simulink subsystem "VehicleElectric"  (R2024b)
settings: Solver=VariableStepAuto  StartTime=0.0  StopTime=10.0  RelTol=1e-3
libraries: nesl_utility x1
Description:
  | Vehicle Electric Architecture
  | 
  | ⚡ Main Features:
  | - Dual motor layout: front motor (EM1) and rear motor (EM2)
  | - Central battery pack supplying HV power to motors and charger
  | - Charger block for external charging interface
  | - Driveline subsystem connects motor torque to wheels
  | - Vehicle-level representation with visual layout
  | 
  | 📤 Outputs: Front/Rear Motor Torque, Battery Power, Driveline Response
  | 
  | 📌 Use Case: Vehicle-level studies of AWD/FWD/RWD configurations, energy flow, and efficiency
settings Model: Creator=jjha  LastModifiedBy=jjha
settings OptimizationCC: ReuseModelBlockBuffer=off
settings RTWCC: GPUComputeCapability=3.5

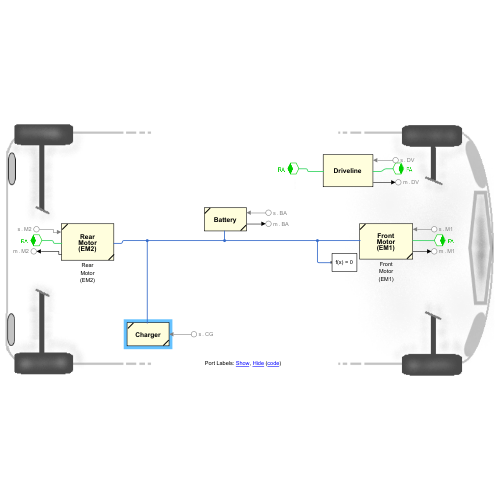
[thumbnail: Simulink's stored preview of the top-level diagram]
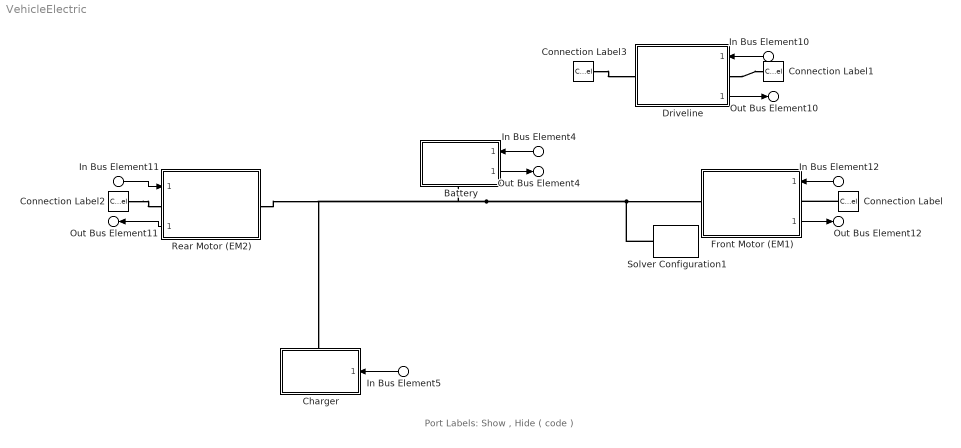
== system VehicleElectric ==
  note: Port Labels: Show , Hide ( code )
  In Bus Element4 : Inport  PortName=s  Element=BA
  In Bus Element10 : Inport  PortName=s  Element=DV
  In Bus Element11 : Inport  PortName=s  Element=M2
  In Bus Element12 : Inport  PortName=s  Element=M1
  In Bus Element5 : Inport  PortName=s  Element=CG
  Battery : Subsystem  ReferencedSubsystem=BatteryLumped
      settings: PortSchema="{\"entries\":[{\"content\":{\"sides\":[{\"content\":{\"connectorIds\":[\"In1\",\"Out1\"]},\"type\":\"ConnectorPlacement.EquallySpacedRectSide\",\"uuid\":\"8937d0fc-2bf4-4b6f-a857-82b384a76c94\"},{\"content\":{\"side\":\"RIGHT\"},\"type\":\"ConnectorPlacement.EquallySpacedRectSide\",\"uuid\":\"1ccbeec6-a013-4076-9f98-cb308866a19c\"},{\"content\":{\"side\":\"TOP\"},\"type\":\"ConnectorPlacement.EquallySpacedRectSide\",\"uuid\":\"77a454e3-c37c-480e-9dd0-9550186f5eb3\"},{\"content\":{\"connectorIds\":[\"RConn1\"],\"side\":\"BOTTOM\"},\"type\":\"ConnectorPlacement.EquallySpacedRectSide\",\"uuid\":\"f9a87c6a-7374-41c2-a5df-89d60c915a70\"}]},\"type\":\"ConnectorPlacement.EquallySpacedConnector\",\"uuid\":\"fe008494-fd6d-45a8-bf6b-36872afbad95\"}],\"packageUris\":[\"http://schema.mathworks.com/mf0/Connector/R2020b\"],\"version\":\"1.0\"}"
  Charger : Subsystem  ReferencedSubsystem=Charger
      settings: PortSchema="{\"entries\":[{\"content\":{\"sides\":[{\"content\":{\"connectorIds\":[\"In1\"]},\"type\":\"ConnectorPlacement.EquallySpacedRectSide\",\"uuid\":\"cb45011f-5d5d-4b7e-92e7-7d115d1e4fd6\"},{\"content\":{\"side\":\"RIGHT\"},\"type\":\"ConnectorPlacement.EquallySpacedRectSide\",\"uuid\":\"cd67087d-6bbf-411e-9f50-cc3c1f5fce85\"},{\"content\":{\"connectorIds\":[\"LConn1\"],\"side\":\"TOP\"},\"type\":\"ConnectorPlacement.EquallySpacedRectSide\",\"uuid\":\"32ff64c9-862a-431f-9f24-2baf455cdab5\"}]},\"type\":\"ConnectorPlacement.EquallySpacedConnector\",\"uuid\":\"13ffd7d0-36a1-4766-a9dc-2d010b2a8713\"}],\"packageUris\":[\"http://schema.mathworks.com/mf0/Connector/R2020b\"],\"version\":\"1.0\"}"
  Connection Label : ConnectionLabel  Label=FA
  Connection Label1 : ConnectionLabel  Label=FA
  Connection Label2 : ConnectionLabel  Label=RA
  Connection Label3 : ConnectionLabel  Label=RA
  Driveline : Subsystem  ReferencedSubsystem=DrivelineWithBraking
      settings: PortSchema="{\"entries\":[{\"content\":{\"sides\":[{\"content\":{\"connectorIds\":[\"In1\",\"LConn1\",\"Out1\"]},\"type\":\"ConnectorPlacement.EquallySpacedRectSide\",\"uuid\":\"f321ff85-78a4-45a4-ab97-f20c5abfaf5e\"},{\"content\":{\"connectorIds\":[\"RConn1\"],\"side\":\"RIGHT\"},\"type\":\"ConnectorPlacement.EquallySpacedRectSide\",\"uuid\":\"2baf3540-3ef2-4140-8c68-0a1895e3ee25\"},{\"content\":{\"side\":\"TOP\"},\"type\":\"ConnectorPlacement.EquallySpacedRectSide\",\"uuid\":\"1e5b09ba-71c5-41d6-b265-2fb2d783e941\"}]},\"type\":\"ConnectorPlacement.EquallySpacedConnector\",\"uuid\":\"4c01441a-ee4a-4858-900a-4caacc6910c3\"}],\"packageUris\":[\"http://schema.mathworks.com/mf0/Connector/R2020b\"],\"version\":\"1.0\"}"
  Front Motor (EM1) : Subsystem  ReferencedSubsystem=MotorDriveGear  max_torque=electricDrive.max_torque  max_power=electricDrive.max_power  Tctc=electricDrive.Tctc  motor_loss_map=electricDrive.motor_loss_map
      settings: PortSchema="{\"entries\":[{\"content\":{\"sides\":[{\"content\":{\"connectorIds\":[\"LConn1\"]},\"type\":\"ConnectorPlacement.EquallySpacedRectSide\",\"uuid\":\"a991d568-7bab-4556-87b6-8d42c862be0a\"},{\"content\":{\"connectorIds\":[\"In1\",\"RConn1\",\"Out1\"],\"side\":\"RIGHT\"},\"type\":\"ConnectorPlacement.EquallySpacedRectSide\",\"uuid\":\"8f8bc0bf-e5c4-4152-82a4-fed810842728\"},{\"content\":{\"side\":\"TOP\"},\"type\":\"ConnectorPlacement.EquallySpacedRectSide\",\"uuid\":\"0a77f6d5-c1ac-4c14-8252-3a4fffbf16b3\"},{\"content\":{\"side\":\"BOTTOM\"},\"type\":\"ConnectorPlacement.EquallySpacedRectSide\",\"uuid\":\"4695f65e-5b66-4095-8b3b-76ce53ac4943\"}]},\"type\":\"ConnectorPlacement.EquallySpacedConnector\",\"uuid\":\"97a94dc1-aa8d-40f4-b132-425677487f87\"}],\"packageUris\":[\"http://schema.mathworks.com/mf0/Connector/R2020b\"],\"version\":\"1.0\"}"
  Rear Motor (EM2) : Subsystem  ReferencedSubsystem=MotorDriveGear  max_torque=electricDrive.max_torque  max_power=electricDrive.max_power  Tctc=electricDrive.Tctc  motor_loss_map=electricDrive.motor_loss_map
      settings: PortSchema="{\"entries\":[{\"content\":{\"sides\":[{\"content\":{\"connectorIds\":[\"In1\",\"RConn1\",\"Out1\"]},\"type\":\"ConnectorPlacement.EquallySpacedRectSide\",\"uuid\":\"a991d568-7bab-4556-87b6-8d42c862be0a\"},{\"content\":{\"connectorIds\":[\"LConn1\"],\"side\":\"RIGHT\"},\"type\":\"ConnectorPlacement.EquallySpacedRectSide\",\"uuid\":\"8f8bc0bf-e5c4-4152-82a4-fed810842728\"},{\"content\":{\"side\":\"TOP\"},\"type\":\"ConnectorPlacement.EquallySpacedRectSide\",\"uuid\":\"0a77f6d5-c1ac-4c14-8252-3a4fffbf16b3\"}]},\"type\":\"ConnectorPlacement.EquallySpacedConnector\",\"uuid\":\"97a94dc1-aa8d-40f4-b132-425677487f87\"}],\"packageUris\":[\"http://schema.mathworks.com/mf0/Connector/R2020b\"],\"version\":\"1.0\"}"
  Solver Configuration1 : nesl_utility/Solver Configuration  PhysicalDomain=network_engine_domain  SubClassName=solver  LeftPortType=input  RightPortType=generic  Tones=[]  Harmonics=[]  SimulateNoise=off  Profile=off  UseLocalSampling=off  EnableSwitchedLinearOptims=on  FrequencyDomain=off  UseCCode=off  RelTol=0.001  AbsTol=0.001  MinStep=1e-09  ToWorkspace=off  RevertToSquareIcSolve=off  NumHomotopyIterations=100  PhasorMode=off  PhasorModeNumHarmonics=1  ConsistencySolver=NEWTON_XTOL_AFTER_FTOL  IndexReductionMethod=DerivativeReplacement  DoDC=off  ResidualTolerance=1e-09  ConsistencyTolSource=GLOBAL  ConsistencyAbsTol=0.001  ConsistencyRelTol=0.001  ConsistencyTolFactor=0.001  UseLocalSolver=off  LocalSolverChoice=NE_BACKWARD_EULER_ADVANCER  ResolveIndetEquations=on  FunctionEvalNumThread=1  LocalSolverSampleTime=0.1  DoFixedCost=off  MaxNonlinIter=3  MaxModeIter=2  ComputeImpulses=off  ImpulseIterations=2  LinearAlgebra=auto  LinearAlgebraNumThread=0  EquationFormulation=NE_TIME_EF  DelaysMemoryBudget=1024  AutomaticFiltering=on  FilteringTimeConstant=0.001  PartitionStorageMethod=AS_NEEDED  PartitionMemoryBudget=1024  PartitionMethod=ROBUST  MultibodyUseLocalSolver=off  MultibodyLocalSolverChoice=ODE1  MultibodyLocalSolverSampleTime=0.001
  Out Bus Element4 : Outport  PortName=m  Element=BA
  Out Bus Element10 : Outport  PortName=m  Element=DV
  Out Bus Element11 : Outport  PortName=m  Element=M2
  Out Bus Element12 : Outport  PortName=m  Element=M1
  wires:
  In Bus Element4/1 -> Battery/1
  Battery/1 -> Out Bus Element4/1
  Driveline/1 -> Out Bus Element10/1
  In Bus Element10/1 -> Driveline/1
  In Bus Element11/1 -> Rear Motor (EM2)/1
  Rear Motor (EM2)/1 -> Out Bus Element11/1
  In Bus Element12/1 -> Front Motor (EM1)/1
  Front Motor (EM1)/1 -> Out Bus Element12/1
  In Bus Element5/1 -> Charger/1
  connections:
  Solver Configuration1/RConn1 -- Charger/LConn1 -- Rear Motor (EM2)/LConn1 -- Battery/RConn1 -- Front Motor (EM1)/LConn1
  Connection Label2/LConn1 -- Rear Motor (EM2)/RConn1
  Connection Label/LConn1 -- Front Motor (EM1)/RConn1
  Driveline/LConn1 -- Connection Label1/LConn1
  Connection Label3/LConn1 -- Driveline/RConn1
